simulink model "MyModel"  (R2024a)
settings: Solver=VariableStepAuto  StartTime=0.0  StopTime=10  MaxStep=0.01  RelTol=1e-3
PreLoadFcn:
  | MyScript
InitFcn:
  | MyScript
undefined symbols (not defined in the file or in its folder): b, k, m, x0
settings Model: NumberOfSteps=10  SnapshotBufferSize=50  SnapshotInterval=50  Creator=ZRAFFAI1  LastModifiedBy=zanga
settings OptimizationCC: OptimizeBlockIOStorage=off
settings HardwareCC: TargetBitPerPointer=64  TargetBitPerSizeT=64  TargetBitPerPtrDiffT=64  TargetLongLongMode=on  TargetIntDivRoundTo=Zero  TargetEndianess=LittleEndian  TargetWordSize=64  TargetHWDeviceType=MATLAB Host  ProdEqTarget=off
settings RTWCC: Description=Rapid Simulation Target  SystemTargetFile=rsim.tlc  GenCodeOnly=on  TemplateMakefile=rsim_default_tmf  GenerateReport=on  LaunchReport=on  RTWCompilerOptimization=on
settings CodeAppCC: ForceParamTrailComments=on  MATLABSourceComments=on
settings RSimTargetCC: TargetLangStandard=C99 (ISO)  InstructionSetFMA=off  OptimizeReductions=off  LogToMDFFile=off

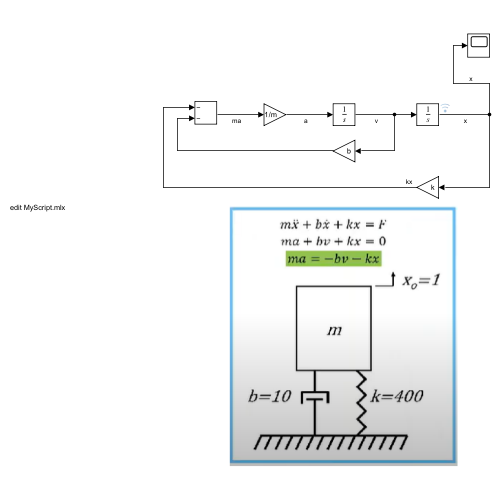
[thumbnail: Simulink's stored preview of the top-level diagram]
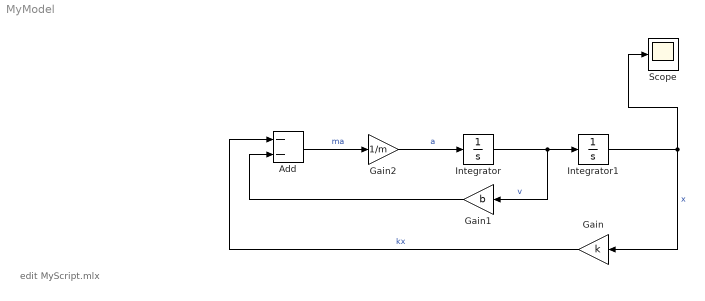
== system MyModel ==
  note: edit MyScript.mlx
  Add : Sum  Inputs=--
  Gain : Gain  Gain=k
  Gain1 : Gain  Gain=b
  Gain2 : Gain  Gain=1/m
  Integrator : Integrator
  Integrator1 : Integrator  InitialCondition=x0
  Scope : Scope
  wires:
  Gain2/1 -> Integrator/1  "a"
  Integrator/1 -> Gain1/1, Integrator1/1  "v"
  Integrator1/1 -> Gain/1, Scope/1  "x"
  Gain/1 -> Add/1  "kx"
  Gain1/1 -> Add/2
  Add/1 -> Gain2/1  "ma"
